simulink model "uas_main_ros2"  (R2026a)
settings: Solver=FixedStepAuto  StopTime=Inf  FixedStep=sample_time
model workspace: external: MAT-File (data not in the file)
values from neighbouring files (symbols this model uses):
  arm_length = 0.17    [uas_parameters.m]
  axes_msg = zeros(1, 124)    [uas_parameters.m]
  button_msg = zeros(1, 124)    [uas_parameters.m]
  drag_coefficient = 0.47    [uas_parameters.m]
  g = 9.81    [PosControllerSystem.m]    (also in uas_parameters.m = 9.80665)
  inertia_xx = 0.007    [uas_parameters.m]
  inertia_yy = 0.007    [uas_parameters.m]
  inertia_zz = 0.012    [uas_parameters.m]
  mass_drone = 0.04    [uas_parameters.m]
  mass_total = 0.04    [PosControllerSystem.m]    (also in uas_parameters.m)
  max_rot_velocity = 838    [uas_parameters.m]
  mix_matrix = inv(motor_constant * allocation_matrix)    [uas_parameters.m]
  moment_constant = 0.016    [uas_parameters.m]
  motor_constant = 8.54858e-06    [uas_parameters.m]
  N = size(waypoints, 1)    [quintic_interp.m]
  reference_area = pi * 75e-3^2    (= 0.0176714586764)    [uas_parameters.m]
  rotor_offset_top = 0.01    [uas_parameters.m]
  route = [0 0 1 ; 9 0 1 ; 9 9 1]    [uas_parameters.m]
  sample_time = 4e-2    (= 0.04)    [uas_parameters.m]
  x0 = 36    [uas_parameters.m]
  y0 = 80    [uas_parameters.m]
  z0 = 1    [uas_parameters.m]
undefined symbols (not defined in the file or in its folder): axes, axes_SL_Info, buttons, buttons_SL_Info, poly_traj, quat2rotm, X, Y, Z
libraries: nesl_utility x32, sm_lib x25, ros2lib x16, dspfdesign x3, simulink x2, sharedtransform x2, sim3dlib x1, uavsim3dlib x1, vrlib x1
(part 3 of 3)

== matlab function uas_main_ros2/quadcopter/quat 2 euler (ROS) ==
  data: q input size=[1 4]; roll_rad output; pitch_rad output; yaw_rad output
function [roll_rad, pitch_rad, yaw_rad] = euler_ros(q)

attitude = quat2eul(q, 'ZYX');

roll_rad = attitude(3);
pitch_rad = attitude(2);
yaw_rad = attitude(1);

== matlab function uas_main_ros2/quadcopter/MATLAB Function ==
  data: u input; y output
function y = get33(u)

y = u(3,3);

== matlab function uas_main_ros2/quadcopter/Subsystem/MATLAB Function1 ==
  data: roll input size=1; pitch input size=1; yaw input size=1; er output size=[3 1]; R input size=[3 3]
function er = lee(roll, pitch, yaw, R)

Rd = eul2rotm([yaw pitch roll], 'ZYX');

P = 1/2 * (Rd.' * R - R.' * Rd) ;

er = [P(3,2) ; P(1,3) ; P(2,1)] ;

== matlab function uas_main_ros2/subscribers1/MATLAB Function ==
  data: pos_world input; x_rel output; eul_angles input; y_rel output; z_rel output; yaw_current output; roll_current output; pitch_current output
function [x_rel, y_rel, z_rel, yaw_current, roll_current, pitch_current] = world_to_start_frame(pos_world, eul_angles)

    persistent x0 y0 z0 yaw0 initialized

    % 1. Initialization: Latch the "Home" values on the first frame ONLY
    if isempty(initialized)
        x0 = pos_world(1);
        y0 = pos_world(2);
        z0 = pos_world(3);
        yaw0 = eul_angles(1); % Grabbing Yaw from the ZYX vector
        initialized = true;
    end

    % 2. Calculate global distance from home
    dx = pos_world(1) - x0;
    dy = pos_world(2) - y0;
    dz = pos_world(3) - z0;

    % 3. Rotate into the drone's starting orientation
    psi = yaw0;

    x_rel =  cos(psi)*dx + sin(psi)*dy;
    y_rel = -sin(psi)*dx + cos(psi)*dy;
    z_rel = dz;
    yaw_current = eul_angles(1);
    roll_current=eul_angles(3);
    pitch_current = eul_angles(2);

end

== matlab function uas_main_ros2/subscribers/MATLAB Function1 ==
  data: aux1 input; armed output
function armed = aux1_to_bool(aux1)
% aux1: numeric value from RC channel
% armed: logical 1 if drone is armed, 0 if disarmed

% Threshold: above 1500 = armed, below = disarmed
armed = aux1 > 1500;
end

== matlab function uas_main_ros2/subscribers1/MATLAB Function1 ==
  data: aux1 input; armed output
function armed = aux1_to_bool(aux1)
% aux1: numeric value from RC channel
% armed: logical 1 if drone is armed, 0 if disarmed

% Threshold: above 1500 = armed, below = disarmed
armed = aux1 > 1500;
end

== matlab function uas_main_ros2/subscribers/MATLAB Function2 ==
  data: pos_world input; x_rel output; eul_angles input; y_rel output; z_rel output; yaw_current output
function [x_rel, y_rel, z_rel, yaw_current] = world_to_start_frame(pos_world, eul_angles)

    persistent x0 y0 z0 yaw0 initialized

    % 1. Initialization: Latch the "Home" values on the first frame ONLY
    if isempty(initialized)
        x0 = pos_world(1);
        y0 = pos_world(2);
        z0 = pos_world(3);
        yaw0 = eul_angles(1); % Grabbing Yaw from the ZYX vector
        initialized = true;
    end

    % 2. Calculate global distance from home
    dx = pos_world(1) - x0;
    dy = pos_world(2) - y0;
    dz = pos_world(3) - z0;

    % 3. Rotate into the drone's starting orientation
    psi = yaw0;

    x_rel =  cos(psi)*dx + sin(psi)*dy;
    y_rel = -sin(psi)*dx + cos(psi)*dy;
    z_rel = dz;
    yaw_current = eul_angles(1);
end

== matlab function uas_main_ros2/subscribers/MATLAB Function3 ==
  data: q_in input; q_out output
function q_out = safeQuat(q_in)
% ROS顺序: [x y z w]

persistent q_last

if isempty(q_last)
    q_last = [1; 0; 0; 0];
end

% 转成MATLAB顺序
q = q_in;

% 检查非法
if any(isnan(q)) || norm(q) < 1e-6
    q = q_last;
else
    q = q / norm(q);
    q_last = q;
end
q_out = q;

== matlab function uas_main_ros2/subscribers1/MATLAB Function2 ==
  data: pos_world input; x_rel output; eul_angles input; y_rel output; z_rel output; yaw_current output
function [x_rel, y_rel, z_rel, yaw_current] = world_to_start_frame(pos_world, eul_angles)

    persistent x0 y0 z0 yaw0 initialized

    % 1. Initialization: Latch the "Home" values on the first frame ONLY
    if isempty(initialized)
        x0 = pos_world(1);
        y0 = pos_world(2);
        z0 = pos_world(3);
        yaw0 = eul_angles(1); % Grabbing Yaw from the ZYX vector
        initialized = true;
    end

    % 2. Calculate global distance from home
    dx = pos_world(1) - x0;
    dy = pos_world(2) - y0;
    dz = pos_world(3) - z0;

    % 3. Rotate into the drone's starting orientation
    psi = yaw0;

    x_rel =  cos(psi)*dx + sin(psi)*dy;
    y_rel = -sin(psi)*dx + cos(psi)*dy;
    z_rel = dz;
    yaw_current = eul_angles(1);
end

== matlab function uas_main_ros2/subscribers1/MATLAB Function3 ==
  data: q_in input; q_out output
function q_out = safeQuat(q_in)
% ROS顺序: [x y z w]

persistent q_last

if isempty(q_last)
    q_last = [1; 0; 0; 0];
end

% 转成MATLAB顺序
q = q_in;

% 检查非法
if any(isnan(q)) || norm(q) < 1e-6
    q = q_last;
else
    q = q / norm(q);
    q_last = q;
end
q_out = q;

== matlab function uas_main_ros2/subscribers/MATLAB Function ==
  data: pos_world input; x_rel output; eul_angles input; y_rel output; z_rel output; yaw_current output; roll_current output; pitch_current output
function [x_rel, y_rel, z_rel, yaw_current, roll_current, pitch_current] = world_to_start_frame(pos_world, eul_angles)

    persistent x0 y0 z0 yaw0 initialized

    % 1. Initialization: Latch the "Home" values on the first frame ONLY
    if isempty(initialized)
        x0 = pos_world(1);
        y0 = pos_world(2);
        z0 = pos_world(3);
        yaw0 = eul_angles(1); % Grabbing Yaw from the ZYX vector
        initialized = true;
    end

    % 2. Calculate global distance from home
    dx = pos_world(1) - x0;
    dy = pos_world(2) - y0;
    dz = pos_world(3) - z0;

    % 3. Rotate into the drone's starting orientation
    psi = yaw0;

    x_rel =  cos(psi)*dx + sin(psi)*dy;
    y_rel = -sin(psi)*dx + cos(psi)*dy;
    z_rel = dz;
    yaw_current = eul_angles(1);
    roll_current=eul_angles(3);
    pitch_current = eul_angles(2);

end

== matlab function uas_main_ros2/position controller/compute_roll_pitch ==
  data: F_d input; roll output; yaw_d input; pitch output
function [roll, pitch] = compute_roll_pitch(F_d, yaw_d)

yaw_dt = yaw_d + pi/2;
uyt = [cos(yaw_dt); sin(yaw_dt); 0];
uz = F_d/norm(F_d);
ux = cross(uyt, uz);
uy = cross(uz, ux);

attitude = rotm2eul([ux uy uz], 'ZYX');

roll = attitude(3);
pitch = attitude(2);

== matlab function uas_main_ros2/quadcopter/quat 2 euler (UE) ==
  data: q input size=[1 4]; attitude output
function attitude = euler_ue(q)

attitude = quat2eul(q, 'ZYX');

attitude = [attitude(1) attitude(2) attitude(3)];

== matlab function uas_main_ros2/quadcopter/position controller/compute_roll_pitch ==
  data: F_d input; roll output; yaw_d input; pitch output
function [roll, pitch] = compute_roll_pitch(F_d, yaw_d)

yaw_dt = yaw_d + pi/2;
uyt = [cos(yaw_dt); sin(yaw_dt); 0];
uz = F_d/norm(F_d);
ux = cross(uyt, uz);
uy = cross(uz, ux);

attitude = rotm2eul([ux uy uz], 'ZYX');

roll = attitude(3);
pitch = attitude(2);

== stateflow chart uas_main_ros2/waypoint navigation (Ex. 6.1 and 7.1) ==
  state go
    pd = [r(i, 1) ; r(i, 2) ; r(i, 3)]
  (default) -> go : {i = 1}
  go -> (junction 26) : [reached(pd, p)]
  (junction 26) -> go : [i < size(r, 1)]{i = i + 1}
  data: setpoint_position function_input; position function_input; is_reached function_output; r input; i local; p input; pd output size=[3 1]
  function is_reached = reached(setpoint_position, position):
    | function is_reached = reached(setpoint_position, position)
    | is_reached = norm(position - setpoint_position) < 0.05;
